simulink model "SVmodulation_exercise_done"  (R2013b)
settings: Solver=ode45  StartTime=0.0  StopTime=0.02*2  FixedStep=1/fs  RelTol=1e-3
undefined symbols (not defined in the file): fs
settings Model: Creator=Fitim k  LastModifiedBy=Fitim k
settings DataIOCC: SignalLoggingSaveFormat=ModelDataLogs
settings OptimizationCC: BlockReduction=off  BooleanDataType=off  InitFltsAndDblsToZero=on
settings DebuggingCC: SaveWithParameterizedLinksMsg=none  SignalResolutionControl=TryResolveAllWithWarning  MultiTaskDSMMsg=warning  MultiTaskCondExecSysMsg=none  FcnCallInpInsideContextMsg=UseLocalSettings
settings RTWCC: IncludeERTFirstTime=on
settings GRTTargetCC: TargetFcnLib=ansi_tfl_tmw.mat  CombineOutputUpdateFcns=off  GRTInterface=on

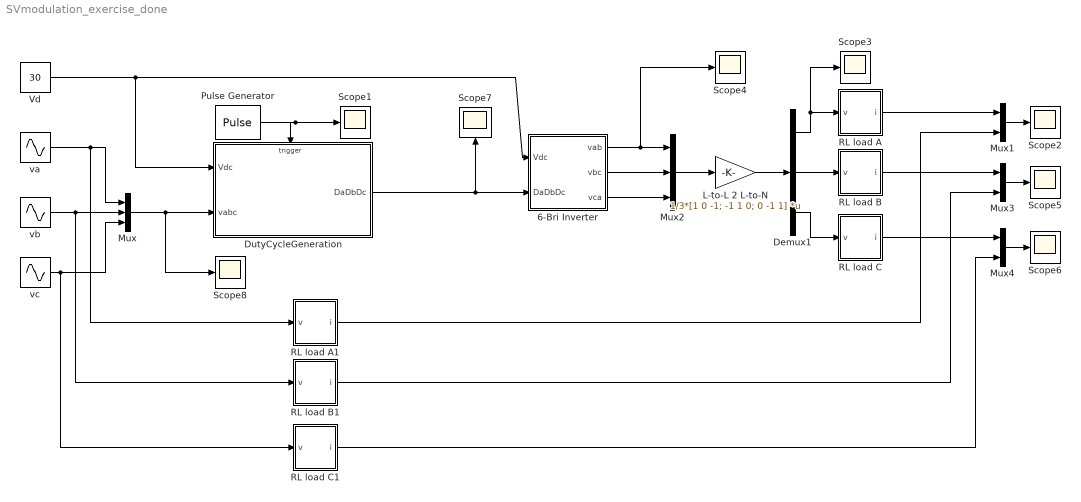
== system SVmodulation_exercise_done ==
  6-Bri Inverter : Subsystem
  Demux1 : Demux  Outputs=3
  DutyCycleGeneration : Subsystem
  L-to-L 2 L-to-N : Gain  Gain=1/3*[1 0 -1; -1 1 0; 0 -1 1]  Multiplication=Matrix(K*u)
  Mux : Mux  Inputs=3
  Mux1 : Mux  Inputs=2
  Mux2 : Mux  Inputs=3
  Mux3 : Mux  Inputs=2
  Mux4 : Mux  Inputs=2
  Pulse Generator : DiscretePulseGenerator  PulseType=Time based  Period=1/fs  PulseWidth=50  PhaseDelay=1/fs/4
  RL load A : Subsystem
  RL load A1 : Subsystem
  RL load B : Subsystem
  RL load B1 : Subsystem
  RL load C : Subsystem
  RL load C1 : Subsystem
  Scope{1..8} (8 alike) : Scope
      Scope1 settings: SaveName=ScopeData4
      Scope2 settings: SaveName=ScopeData9
      Scope3 settings: SaveName=ScopeData10
      Scope4 settings: SaveName=ScopeData11
      Scope5 settings: SaveName=ScopeData12
      Scope6 settings: SaveName=ScopeData13
      Scope8 settings: SaveName=ScopeData14
  Vd : Constant  Value=30
  va : Sin  Amplitude=10  Frequency=2*pi*50  Phase=pi/2  SampleTime=0
  vb : Sin  Amplitude=10  Frequency=2*pi*50  Phase=-2*pi/3+pi/2  SampleTime=0
  vc : Sin  Amplitude=10  Frequency=2*pi*50  Phase=+2*pi/3+pi/2  SampleTime=0
  wires:
  va/1 -> Mux/1, RL load A1/1(v)
  vb/1 -> Mux/2, RL load B1/1(v)
  vc/1 -> Mux/3, RL load C1/1(v)
  Mux/1 -> DutyCycleGeneration/2(vabc), Scope8/1
  Vd/1 -> DutyCycleGeneration/1(Vdc), 6-Bri Inverter/1(Vdc)
  DutyCycleGeneration/1(DaDbDc) -> Scope7/1, 6-Bri Inverter/2(DaDbDc)
  Pulse Generator/1 -> DutyCycleGeneration/Trigger, Scope1/1
  L-to-L 2 L-to-N/1 -> Demux1/1
  6-Bri Inverter/1(vab) -> Mux2/1, Scope4/1
  6-Bri Inverter/2(vbc) -> Mux2/2
  6-Bri Inverter/3(vca) -> Mux2/3
  Mux2/1 -> L-to-L 2 L-to-N/1
  Demux1/1 -> RL load A/1(v), Scope3/1
  Demux1/2 -> RL load B/1(v)
  Demux1/3 -> RL load C/1(v)
  RL load A/1(i) -> Mux1/1
  RL load B/1(i) -> Mux3/1
  RL load C/1(i) -> Mux4/1
  RL load A1/1(i) -> Mux1/2
  RL load B1/1(i) -> Mux3/2
  RL load C1/1(i) -> Mux4/2
  Mux1/1 -> Scope2/1
  Mux3/1 -> Scope5/1
  Mux4/1 -> Scope6/1

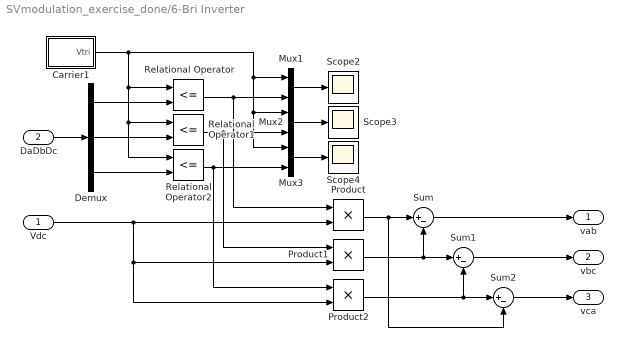
== system SVmodulation_exercise_done/6-Bri Inverter ==
  Vdc : Inport
  DaDbDc : Inport  Port=2
  Carrier1 : Subsystem  mask{fsw=fs}
      mask prompts: fsw "switching frequency"
      mask init:
      | fsw2=fsw*2;
      | x=[0 1/4 3/4 1];
      | y=[0 -1     1    0];
      mask Display: plot([x  x+1 ],[y y])
  Demux : Demux  Outputs=3
  Mux1 : Mux  Inputs=2
  Mux2 : Mux  Inputs=2
  Mux3 : Mux  Inputs=2
  Product : Product  RndMeth=Zero
  Product1 : Product  RndMeth=Zero
  Product2 : Product  RndMeth=Zero
  Relational Operator : RelationalOperator  Operator=<=
  Relational Operator1 : RelationalOperator  Operator=<=
  Relational Operator2 : RelationalOperator  Operator=<=
  Scope2 : Scope
      settings: SaveName=ScopeData5
  Scope3 : Scope
      settings: SaveName=ScopeData7
  Scope4 : Scope
      settings: SaveName=ScopeData8
  Sum : Sum  Inputs=|+-
  Sum1 : Sum  Inputs=|+-
  Sum2 : Sum  Inputs=|+-
  vab : Outport
  vbc : Outport  Port=2
  vca : Outport  Port=3
  wires:
  Demux/1 -> Relational Operator/2
  Carrier1/1(Vtri) -> Relational Operator/1, Relational Operator1/1, Relational Operator2/1, Mux1/1, Mux3/1, Mux2/1
  Mux1/1 -> Scope2/1
  Relational Operator/1 -> Mux1/2, Product/1
  Demux/2 -> Relational Operator1/2
  Demux/3 -> Relational Operator2/2
  Mux2/1 -> Scope3/1
  Mux3/1 -> Scope4/1
  Relational Operator1/1 -> Mux2/2, Product1/1
  Relational Operator2/1 -> Mux3/2, Product2/1
  DaDbDc/1 -> Demux/1
  Vdc/1 -> Product/2, Product1/2, Product2/2
  Product/1 -> Sum/1, Sum2/2
  Product1/1 -> Sum/2, Sum1/1
  Product2/1 -> Sum1/2, Sum2/1
  Sum/1 -> vab/1
  Sum1/1 -> vbc/1
  Sum2/1 -> vca/1

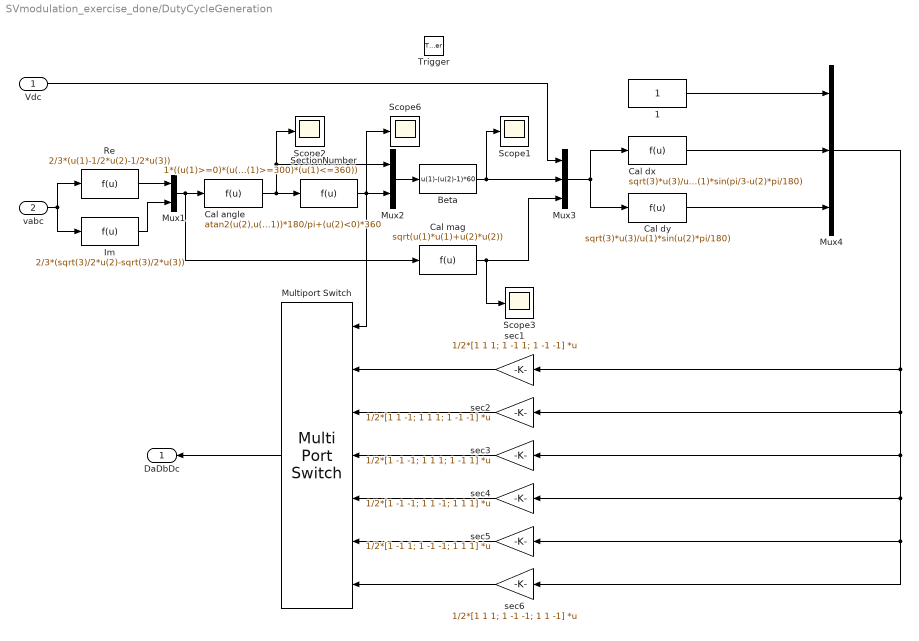
== system SVmodulation_exercise_done/DutyCycleGeneration ==
  Vdc : Inport
  vabc : Inport  Port=2
  Trigger : TriggerPort
  1 : Constant
  Beta : Fcn  Expr=u(1)-(u(2)-1)*60
  Cal angle : Fcn  Expr=atan2(u(2),u(1))*180/pi+(u(2)<0)*360
  Cal dx : Fcn  Expr=sqrt(3)*u(3)/u(1)*sin(pi/3-u(2)*pi/180)
  Cal dy : Fcn  Expr=sqrt(3)*u(3)/u(1)*sin(u(2)*pi/180)
  "Cal mag " : Fcn  Expr=sqrt(u(1)*u(1)+u(2)*u(2))
  Im : Fcn  Expr=2/3*(sqrt(3)/2*u(2)-sqrt(3)/2*u(3))
  Multiport Switch : MultiPortSwitch  Inputs=6
  Mux1 : Mux  Inputs=2
  Mux2 : Mux  Inputs=2
  Mux3 : Mux  Inputs=3
  Mux4 : Mux  Inputs=3
  Re : Fcn  Expr=2/3*(u(1)-1/2*u(2)-1/2*u(3))
  Scope{1..3,6} (4 alike) : Scope
      Scope2 settings: SaveName=ScopeData2
      Scope3 settings: SaveName=ScopeData3
      Scope6 settings: SaveName=ScopeData6
  SectionNumber : Fcn  Expr=1*((u(1)>=0)*(u(1)<60))+2*((u(1)>=60)*(u(1)<120))+3*((u(1)>=120)*(u(1)<180))+4*((u(1)>=180)*(u(1)<240))+5*((u(1)>=240)*(u(1)<300))+6*((u(1)>=300)*(u(1)<=360))
  sec1 : Gain  Gain=1/2*[1 1 1; 1 -1 1; 1 -1 -1]  Multiplication=Matrix(K*u)
  sec2 : Gain  Gain=1/2*[1 1 -1; 1 1 1; 1 -1 -1]  Multiplication=Matrix(K*u)
  sec3 : Gain  Gain=1/2*[1 -1 -1; 1 1 1; 1 -1 1]  Multiplication=Matrix(K*u)
  sec4 : Gain  Gain=1/2*[1 -1 -1; 1 1 -1; 1 1 1]  Multiplication=Matrix(K*u)
  sec5 : Gain  Gain=1/2*[1 -1 1; 1 -1 -1; 1 1 1]  Multiplication=Matrix(K*u)
  sec6 : Gain  Gain=1/2*[1 1 1; 1 -1 -1; 1 1 -1]  Multiplication=Matrix(K*u)
  DaDbDc : Outport
  wires:
  Re/1 -> Mux1/1
  Im/1 -> Mux1/2
  Mux1/1 -> Cal angle/1, "Cal mag "/1
  Cal angle/1 -> SectionNumber/1, Mux2/1, Scope2/1
  SectionNumber/1 -> Mux2/2, Scope6/1, Multiport Switch/1
  Mux2/1 -> Beta/1
  Beta/1 -> Mux3/2, Scope1/1
  "Cal mag "/1 -> Mux3/3, Scope3/1
  Mux3/1 -> Cal dx/1, Cal dy/1
  Cal dx/1 -> Mux4/2
  Cal dy/1 -> Mux4/3
  Mux4/1 -> sec1/1, sec2/1, sec3/1, sec4/1, sec5/1, sec6/1
  sec1/1 -> Multiport Switch/2
  Multiport Switch/1 -> DaDbDc/1
  1/1 -> Mux4/1
  sec2/1 -> Multiport Switch/3
  sec3/1 -> Multiport Switch/4
  sec4/1 -> Multiport Switch/5
  sec5/1 -> Multiport Switch/6
  sec6/1 -> Multiport Switch/7
  vabc/1 -> Im/1, Re/1
  Vdc/1 -> Mux3/1

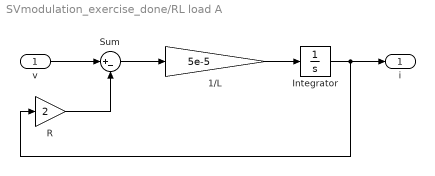
== system SVmodulation_exercise_done/RL load A ==
  v : Inport
  1/L : Gain  Gain=5e-5
  Integrator : Integrator
  R : Gain  Gain=2
  Sum : Sum  Inputs=|+-
  i : Outport
  wires:
  R/1 -> Sum/2
  Sum/1 -> 1/L/1
  1/L/1 -> Integrator/1
  Integrator/1 -> R/1, i/1
  v/1 -> Sum/1

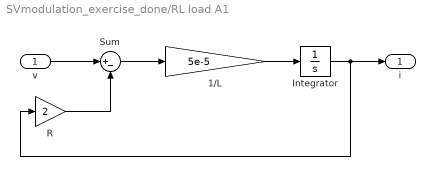
== system SVmodulation_exercise_done/RL load A1 ==
  v : Inport
  1/L : Gain  Gain=5e-5
  Integrator : Integrator
  R : Gain  Gain=2
  Sum : Sum  Inputs=|+-
  i : Outport
  wires:
  v/1 -> Sum/1
  Integrator/1 -> i/1, R/1
  1/L/1 -> Integrator/1
  Sum/1 -> 1/L/1
  R/1 -> Sum/2

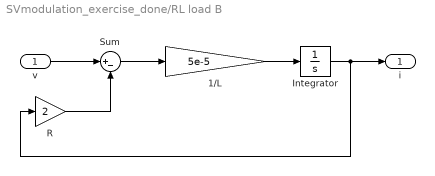
== system SVmodulation_exercise_done/RL load B ==
  v : Inport
  1/L : Gain  Gain=5e-5
  Integrator : Integrator
  R : Gain  Gain=2
  Sum : Sum  Inputs=|+-
  i : Outport
  wires:
  v/1 -> Sum/1
  Integrator/1 -> i/1, R/1
  1/L/1 -> Integrator/1
  Sum/1 -> 1/L/1
  R/1 -> Sum/2

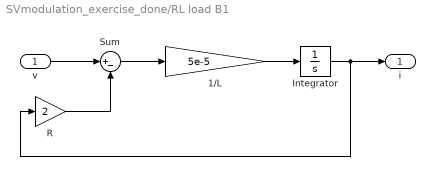
== system SVmodulation_exercise_done/RL load B1 ==
  v : Inport
  1/L : Gain  Gain=5e-5
  Integrator : Integrator
  R : Gain  Gain=2
  Sum : Sum  Inputs=|+-
  i : Outport
  wires:
  R/1 -> Sum/2
  Sum/1 -> 1/L/1
  1/L/1 -> Integrator/1
  Integrator/1 -> R/1, i/1
  v/1 -> Sum/1

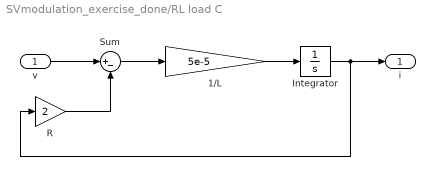
== system SVmodulation_exercise_done/RL load C ==
  v : Inport
  1/L : Gain  Gain=5e-5
  Integrator : Integrator
  R : Gain  Gain=2
  Sum : Sum  Inputs=|+-
  i : Outport
  wires:
  v/1 -> Sum/1
  Integrator/1 -> i/1, R/1
  1/L/1 -> Integrator/1
  Sum/1 -> 1/L/1
  R/1 -> Sum/2

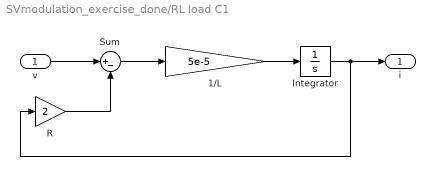
== system SVmodulation_exercise_done/RL load C1 ==
  v : Inport
  1/L : Gain  Gain=5e-5
  Integrator : Integrator
  R : Gain  Gain=2
  Sum : Sum  Inputs=|+-
  i : Outport
  wires:
  R/1 -> Sum/2
  Sum/1 -> 1/L/1
  1/L/1 -> Integrator/1
  Integrator/1 -> R/1, i/1
  v/1 -> Sum/1

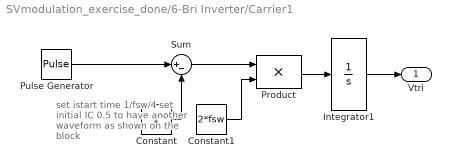
== system SVmodulation_exercise_done/6-Bri Inverter/Carrier1 ==
  note: set istart time 1/fsw/4
      | set initial IC 0.5
      | to have another waveform
      |  as shown on the block
  Constant : Constant
  Constant1 : Constant  Value=2*fsw
  Integrator1 : Integrator
  Product : Product  SaturateOnIntegerOverflow=on  OutDataTypeStr=Inherit: Same as first input
  Pulse Generator : DiscretePulseGenerator  PulseType=Time based  Amplitude=2  Period=1/fsw  PulseWidth=50
  Sum : Sum  Inputs=|+-  SaturateOnIntegerOverflow=on
  Vtri : Outport  InitialOutput=0
  wires:
  Pulse Generator/1 -> Sum/1
  Constant/1 -> Sum/2
  Sum/1 -> Product/1
  Constant1/1 -> Product/2
  Product/1 -> Integrator1/1
  Integrator1/1 -> Vtri/1
